simulink model "oversample2x_2samples_per_clock"  (R2016b)
settings: Solver=VariableStepAuto  StartTime=0.0  StopTime=samples_per_channel*number_channels  RelTol=1e-3
PreLoadFcn:
  | setup
values from neighbouring files (symbols this model uses):
  filts = reshape(filt,number_subband,taps_per_chan)    [setup.m]
undefined symbols (not defined in the file or in its folder): j
libraries: dspxfrm3 x8, dspsigops x2
settings Model: Creator=mdewart  LastModifiedBy=mdewart

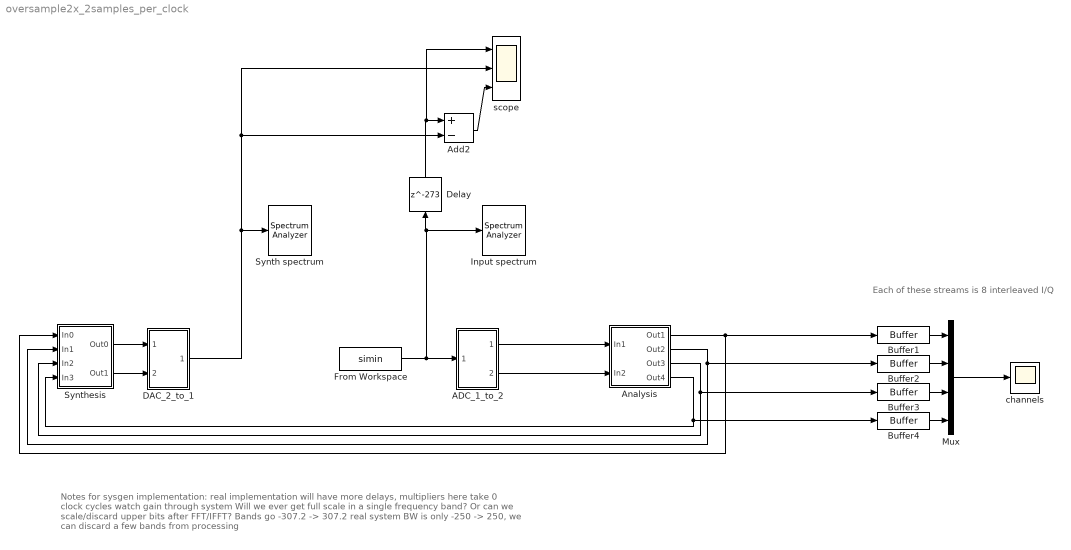
== system oversample2x_2samples_per_clock ==
  note: Notes for sysgen implementation:
      |
      | real implementation will have more delays, multipliers here take 0 clock cycles
      |
      | watch gain through system
      |      Will we ever get full scale in a single frequency band?  Or can we scale/discard upper bits after FFT/IFFT?
      |
      | Bands go -307.2 -> 307.2  real system BW is only -250 -> 250, we can discard a few bands from processing
  note: Each of these streams is 8 interleaved I/Q
  ADC_1_to_2 : Subsystem
  Add2 : Sum  Inputs=+-
  Analysis : Subsystem
  Buffer{1..4} (4 alike) : Buffer  N=8  TreatMby1Signals=One channel  OutputFrames=off
  DAC_2_to_1 : Subsystem
  Delay : Delay  DelayLength=273  InitialCondition=0
  From Workspace : FromWorkspace  VariableName=simin  SampleTime=1  Interpolate=off  OutputAfterFinalValue=Cyclic repetition
  Input spectrum : SpectrumAnalyzer
  Mux : Mux
  Synth spectrum : SpectrumAnalyzer
  Synthesis : Subsystem
  channels : Scope
  scope : Scope  NumInputPorts=3
  wires:
  Synthesis/1(Out0) -> DAC_2_to_1/1(In1)
  Synthesis/2(Out1) -> DAC_2_to_1/2(In2)
  ADC_1_to_2/1(Out1) -> Analysis/1(In1)
  ADC_1_to_2/2(Out2) -> Analysis/2(In2)
  Analysis/4(Out4) -> Buffer4/1, Synthesis/4(In3)
  Analysis/3(Out3) -> Buffer3/1, Synthesis/3(In2)
  Analysis/2(Out2) -> Buffer2/1, Synthesis/2(In1)
  Analysis/1(Out1) -> Buffer1/1, Synthesis/1(In0)
  From Workspace/1 -> Delay/1, Input spectrum/1, ADC_1_to_2/1(In1)
  Mux/1 -> channels/1
  Buffer1/1 -> Mux/1
  Buffer2/1 -> Mux/2
  Buffer3/1 -> Mux/3
  Buffer4/1 -> Mux/4
  Add2/1 -> scope/3
  DAC_2_to_1/1(Out1) -> Add2/2, scope/2, Synth spectrum/1
  Delay/1 -> Add2/1, scope/1

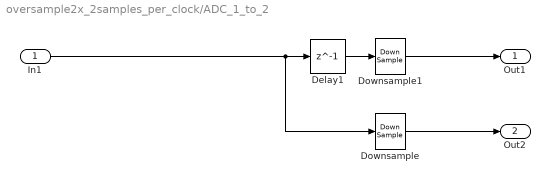
== system oversample2x_2samples_per_clock/ADC_1_to_2 ==
  In1 : Inport
  Delay1 : Delay  DelayLength=1  InitialCondition=0
  Downsample : DownSample  RateOptions=Allow multirate processing
  Downsample1 : DownSample  RateOptions=Allow multirate processing
  Out1 : Outport
  Out2 : Outport  Port=2
  wires:
  Downsample/1 -> Out2/1
  In1/1 -> Downsample/1, Delay1/1
  Downsample1/1 -> Out1/1
  Delay1/1 -> Downsample1/1

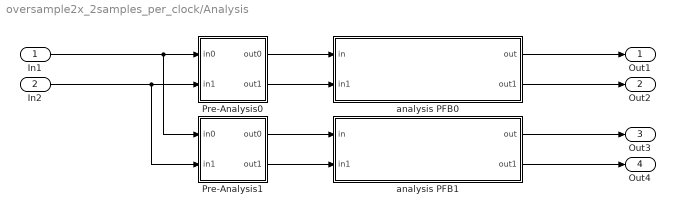
== system oversample2x_2samples_per_clock/Analysis ==
  In1 : Inport
  In2 : Inport  Port=2
  Pre-Analysis0 : Subsystem
  Pre-Analysis1 : Subsystem
  analysis PFB0 : Subsystem
  analysis PFB1 : Subsystem
  Out1 : Outport
  Out2 : Outport  Port=2
  Out3 : Outport  Port=3
  Out4 : Outport  Port=4
  wires:
  analysis PFB0/1(out) -> Out1/1
  analysis PFB1/1(out) -> Out3/1
  Pre-Analysis1/2(out1) -> analysis PFB1/2(in1)
  Pre-Analysis1/1(out0) -> analysis PFB1/1(in)
  Pre-Analysis0/1(out0) -> analysis PFB0/1(in)
  Pre-Analysis0/2(out1) -> analysis PFB0/2(in1)
  analysis PFB1/2(out1) -> Out4/1
  In1/1 -> Pre-Analysis1/1(in0), Pre-Analysis0/1(in0)
  In2/1 -> Pre-Analysis1/2(in1), Pre-Analysis0/2(in1)
  analysis PFB0/2(out1) -> Out2/1

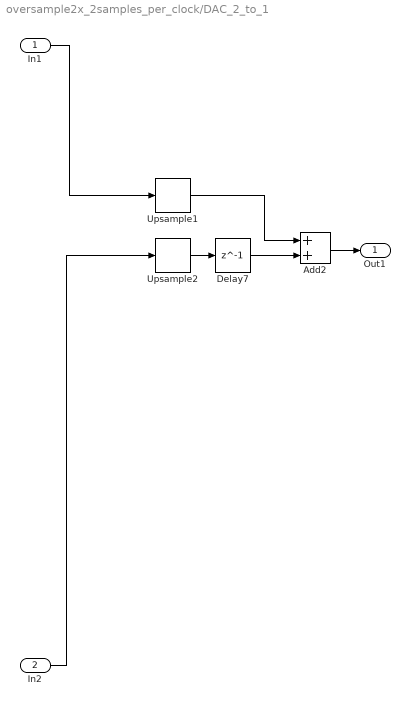
== system oversample2x_2samples_per_clock/DAC_2_to_1 ==
  In1 : Inport
  In2 : Inport  Port=2
  Add2 : Sum
  Delay7 : Delay  DelayLength=1  InitialCondition=0
  Upsample1 : dspsigops/Upsample  N=2  phase=0  RateOptions=Allow multirate processing  ic=0  mode=Unused parameter value
  Upsample2 : dspsigops/Upsample  N=2  phase=0  RateOptions=Allow multirate processing  ic=0  mode=Unused parameter value
  Out1 : Outport
  wires:
  In2/1 -> Upsample2/1
  Delay7/1 -> Add2/2
  In1/1 -> Upsample1/1
  Upsample1/1 -> Add2/1
  Add2/1 -> Out1/1
  Upsample2/1 -> Delay7/1

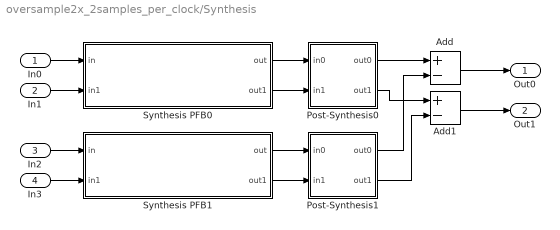
== system oversample2x_2samples_per_clock/Synthesis ==
  In0 : Inport
  In1 : Inport  Port=2
  In2 : Inport  Port=3
  In3 : Inport  Port=4
  Add : Sum  Inputs=+-
  Add1 : Sum  Inputs=+-
  Post-Synthesis0 : Subsystem
  Post-Synthesis1 : Subsystem
  Synthesis PFB0 : Subsystem
  Synthesis PFB1 : Subsystem
  Out0 : Outport
  Out1 : Outport  Port=2
  wires:
  In2/1 -> Synthesis PFB1/1(in)
  In1/1 -> Synthesis PFB0/2(in1)
  In0/1 -> Synthesis PFB0/1(in)
  In3/1 -> Synthesis PFB1/2(in1)
  Synthesis PFB0/2(out1) -> Post-Synthesis0/2(in1)
  Synthesis PFB0/1(out) -> Post-Synthesis0/1(in0)
  Post-Synthesis0/1(out0) -> Add/1
  Post-Synthesis1/1(out0) -> Add/2
  Add/1 -> Out0/1
  Post-Synthesis0/2(out1) -> Add1/1
  Add1/1 -> Out1/1
  Synthesis PFB1/2(out1) -> Post-Synthesis1/2(in1)
  Post-Synthesis1/2(out1) -> Add1/2
  Synthesis PFB1/1(out) -> Post-Synthesis1/1(in0)

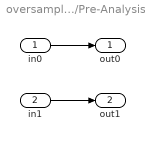
== system oversample2x_2samples_per_clock/Analysis/Pre-Analysis0 ==
  in0 : Inport
  in1 : Inport  Port=2
  out0 : Outport
  out1 : Outport  Port=2
  wires:
  in1/1 -> out1/1
  in0/1 -> out0/1

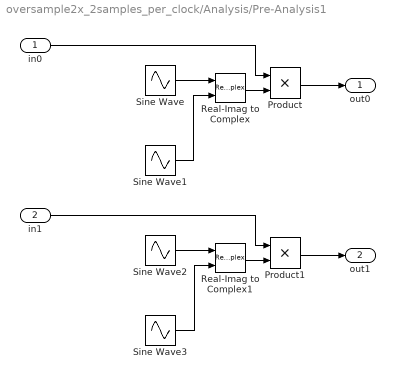
== system oversample2x_2samples_per_clock/Analysis/Pre-Analysis1 ==
  in0 : Inport
  in1 : Inport  Port=2
  Product : Product
  Product1 : Product
  Real-Imag to Complex : RealImagToComplex
  Real-Imag to Complex1 : RealImagToComplex
  Sine Wave : Sin  Frequency=2*pi/32  Phase=-pi/2  SampleTime=2
  Sine Wave1 : Sin  Frequency=2*pi/32  SampleTime=2
  Sine Wave2 : Sin  Frequency=2*pi/32  Phase=-pi/2+pi/16  SampleTime=2
  Sine Wave3 : Sin  Frequency=2*pi/32  Phase=0+pi/16  SampleTime=2
  out0 : Outport
  out1 : Outport  Port=2
  wires:
  in0/1 -> Product/1
  Product/1 -> out0/1
  Product1/1 -> out1/1
  Sine Wave/1 -> Real-Imag to Complex/1
  Sine Wave1/1 -> Real-Imag to Complex/2
  in1/1 -> Product1/1
  Sine Wave2/1 -> Real-Imag to Complex1/1
  Sine Wave3/1 -> Real-Imag to Complex1/2
  Real-Imag to Complex1/1 -> Product1/2
  Real-Imag to Complex/1 -> Product/2

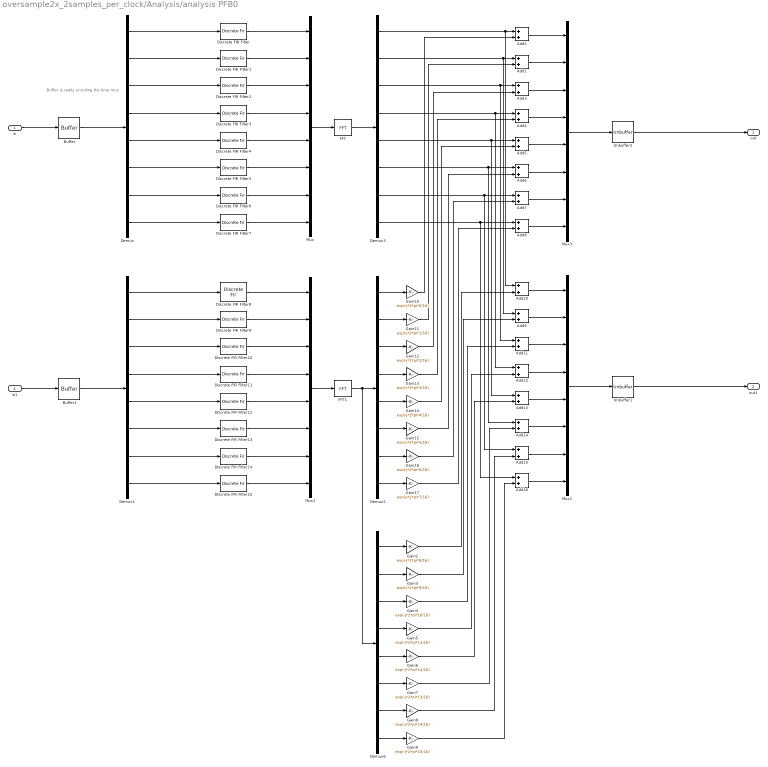
== system oversample2x_2samples_per_clock/Analysis/analysis PFB0 ==
  note: Buffer is really unrolling the time mux
  in : Inport
  in1 : Inport  Port=2
  Add{1..16} (16 alike) : Sum
  Buffer : Buffer  N=8  TreatMby1Signals=One channel  OutputFrames=off
  Buffer1 : Buffer  N=8  TreatMby1Signals=One channel  OutputFrames=off
  Demux{,1..3,6} (5 alike) : Demux  Outputs=8
  Discrete FIR Filter : DiscreteFir  Coefficients=fliplr(filts(1,:))
  Discrete FIR Filter1 : DiscreteFir  Coefficients=fliplr(filts(3,:))
  Discrete FIR Filter10 : DiscreteFir  Coefficients=fliplr(filts(6,:))
  Discrete FIR Filter11 : DiscreteFir  Coefficients=fliplr(filts(8,:))
  Discrete FIR Filter12 : DiscreteFir  Coefficients=fliplr(filts(10,:))
  Discrete FIR Filter13 : DiscreteFir  Coefficients=fliplr(filts(12,:))
  Discrete FIR Filter14 : DiscreteFir  Coefficients=fliplr(filts(14,:))
  Discrete FIR Filter15 : DiscreteFir  Coefficients=fliplr(filts(16,:))
  Discrete FIR Filter2 : DiscreteFir  Coefficients=fliplr(filts(5,:))
  Discrete FIR Filter3 : DiscreteFir  Coefficients=fliplr(filts(7,:))
  Discrete FIR Filter4 : DiscreteFir  Coefficients=fliplr(filts(9,:))
  Discrete FIR Filter5 : DiscreteFir  Coefficients=fliplr(filts(11,:))
  Discrete FIR Filter6 : DiscreteFir  Coefficients=fliplr(filts(13,:))
  Discrete FIR Filter7 : DiscreteFir  Coefficients=fliplr(filts(15,:))
  Discrete FIR Filter8 : DiscreteFir  Coefficients=fliplr(filts(2,:))
  Discrete FIR Filter9 : DiscreteFir  Coefficients=fliplr(filts(4,:))
  FFT : dspxfrm3/FFT  FFTImplementation=Auto  CompMethod=Table lookup  TableOpt=NEW  TableOptActive=Speed  BitRevOrder=off  Normalize=off  InheritFFTLength=on  FFTLength=64  WrapInput=on  roundingMode=Floor  overflowMode=off  firstCoeffDataTypeStr=Inherit: Same word length as input  firstCoeffLastDataTypeStr=Inherit: Same word length as input  outputMin=[]  outputMax=[]
  FFT1 : dspxfrm3/FFT  FFTImplementation=Auto  CompMethod=Table lookup  TableOpt=NEW  TableOptActive=Speed  BitRevOrder=off  Normalize=off  InheritFFTLength=on  FFTLength=64  WrapInput=on  roundingMode=Floor  overflowMode=off  firstCoeffDataTypeStr=Inherit: Same word length as input  firstCoeffLastDataTypeStr=Inherit: Same word length as input  outputMin=[]  outputMax=[]
  Gain10 : Gain  Gain=exp(-j*2*pi*0/16)
  Gain11 : Gain  Gain=exp(-j*2*pi*1/16)
  Gain12 : Gain  Gain=exp(-j*2*pi*2/16)
  Gain13 : Gain  Gain=exp(-j*2*pi*3/16)
  Gain14 : Gain  Gain=exp(-j*2*pi*4/16)
  Gain15 : Gain  Gain=exp(-j*2*pi*5/16)
  Gain16 : Gain  Gain=exp(-j*2*pi*6/16)
  Gain17 : Gain  Gain=exp(-j*2*pi*7/16)
  Gain2 : Gain  Gain=exp(-j*2*pi*8/16)
  Gain3 : Gain  Gain=exp(-j*2*pi*9/16)
  Gain4 : Gain  Gain=exp(-j*2*pi*10/16)
  Gain5 : Gain  Gain=exp(-j*2*pi*11/16)
  Gain6 : Gain  Gain=exp(-j*2*pi*12/16)
  Gain7 : Gain  Gain=exp(-j*2*pi*13/16)
  Gain8 : Gain  Gain=exp(-j*2*pi*14/16)
  Gain9 : Gain  Gain=exp(-j*2*pi*15/16)
  Mux{,1..3} (4 alike) : Mux  Inputs=8
  Unbuffer1 : Unbuffer  SampleBasedProcessing=Same as frame based
  Unbuffer2 : Unbuffer  SampleBasedProcessing=Same as frame based
  out : Outport
  out1 : Outport  Port=2
  wires:
  Add16/1 -> Mux2/8
  Add15/1 -> Mux2/7
  Demux2/2 -> Gain11/1
  Demux2/6 -> Gain15/1
  Demux2/3 -> Gain12/1
  Demux2/5 -> Gain14/1
  Demux2/1 -> Gain10/1
  Demux2/8 -> Gain17/1
  Demux2/7 -> Gain16/1
  Demux2/4 -> Gain13/1
  Mux1/1 -> FFT1/1
  Demux1/4 -> Discrete FIR Filter11/1
  Discrete FIR Filter14/1 -> Mux1/7
  Discrete FIR Filter11/1 -> Mux1/4
  Discrete FIR Filter9/1 -> Mux1/2
  Discrete FIR Filter10/1 -> Mux1/3
  Discrete FIR Filter12/1 -> Mux1/5
  Discrete FIR Filter8/1 -> Mux1/1
  Discrete FIR Filter13/1 -> Mux1/6
  Demux1/6 -> Discrete FIR Filter13/1
  Demux1/1 -> Discrete FIR Filter8/1
  Demux1/3 -> Discrete FIR Filter10/1
  Demux1/8 -> Discrete FIR Filter15/1
  Demux1/5 -> Discrete FIR Filter12/1
  Demux1/7 -> Discrete FIR Filter14/1
  Demux1/2 -> Discrete FIR Filter9/1
  Discrete FIR Filter15/1 -> Mux1/8
  Mux/1 -> FFT/1
  Demux/4 -> Discrete FIR Filter3/1
  Discrete FIR Filter6/1 -> Mux/7
  Discrete FIR Filter3/1 -> Mux/4
  Discrete FIR Filter1/1 -> Mux/2
  Discrete FIR Filter2/1 -> Mux/3
  Discrete FIR Filter4/1 -> Mux/5
  Discrete FIR Filter/1 -> Mux/1
  Discrete FIR Filter5/1 -> Mux/6
  Demux/6 -> Discrete FIR Filter5/1
  Demux/1 -> Discrete FIR Filter/1
  Demux/3 -> Discrete FIR Filter2/1
  Demux/8 -> Discrete FIR Filter7/1
  Demux/5 -> Discrete FIR Filter4/1
  Demux/7 -> Discrete FIR Filter6/1
  Demux/2 -> Discrete FIR Filter1/1
  Buffer/1 -> Demux/1
  Discrete FIR Filter7/1 -> Mux/8
  Buffer1/1 -> Demux1/1
  Mux2/1 -> Unbuffer1/1
  Unbuffer2/1 -> out/1
  FFT/1 -> Demux3/1
  Demux3/8 -> Add16/1, Add8/1
  Demux3/7 -> Add15/1, Add7/1
  Demux3/6 -> Add14/1, Add6/1
  Demux3/5 -> Add13/1, Add5/1
  Demux3/4 -> Add12/1, Add4/1
  Demux3/3 -> Add11/1, Add3/1
  Demux3/2 -> Add9/1, Add1/1
  Demux3/1 -> Add10/1, Add2/1
  Add2/1 -> Mux3/1
  Add1/1 -> Mux3/2
  Add5/1 -> Mux3/5
  Add6/1 -> Mux3/6
  Add3/1 -> Mux3/3
  Add7/1 -> Mux3/7
  Add4/1 -> Mux3/4
  Add8/1 -> Mux3/8
  Mux3/1 -> Unbuffer2/1
  in/1 -> Buffer/1
  Add10/1 -> Mux2/1
  Add11/1 -> Mux2/3
  Add12/1 -> Mux2/4
  Add13/1 -> Mux2/5
  Add14/1 -> Mux2/6
  Add9/1 -> Mux2/2
  Unbuffer1/1 -> out1/1
  Gain10/1 -> Add2/2
  Gain11/1 -> Add1/2
  Gain12/1 -> Add3/2
  Gain13/1 -> Add4/2
  Gain14/1 -> Add5/2
  Gain15/1 -> Add6/2
  Gain16/1 -> Add7/2
  Gain17/1 -> Add8/2
  Demux6/2 -> Gain3/1
  Demux6/6 -> Gain7/1
  Demux6/3 -> Gain4/1
  Demux6/5 -> Gain6/1
  Demux6/1 -> Gain2/1
  Demux6/8 -> Gain9/1
  Demux6/7 -> Gain8/1
  Demux6/4 -> Gain5/1
  FFT1/1 -> Demux6/1, Demux2/1
  Gain2/1 -> Add10/2
  Gain3/1 -> Add9/2
  Gain4/1 -> Add11/2
  Gain5/1 -> Add12/2
  Gain6/1 -> Add13/2
  Gain7/1 -> Add14/2
  Gain8/1 -> Add15/2
  Gain9/1 -> Add16/2
  in1/1 -> Buffer1/1

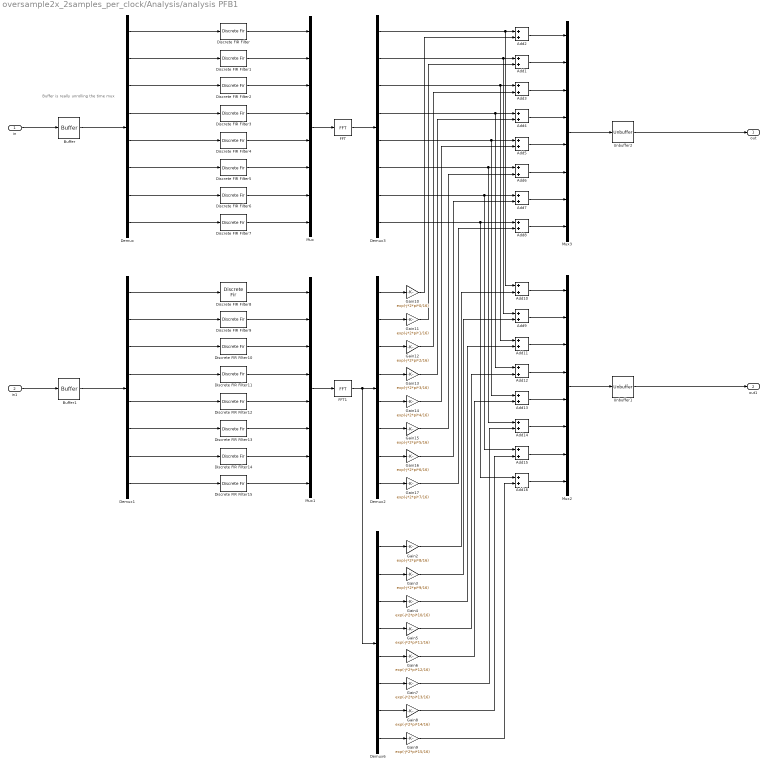
== system oversample2x_2samples_per_clock/Analysis/analysis PFB1 ==
  note: Buffer is really unrolling the time mux
  in : Inport
  in1 : Inport  Port=2
  Add{1..16} (16 alike) : Sum
  Buffer : Buffer  N=8  TreatMby1Signals=One channel  OutputFrames=off
  Buffer1 : Buffer  N=8  TreatMby1Signals=One channel  OutputFrames=off
  Demux{,1..3,6} (5 alike) : Demux  Outputs=8
  Discrete FIR Filter : DiscreteFir  Coefficients=fliplr(filts(1,:))
  Discrete FIR Filter1 : DiscreteFir  Coefficients=fliplr(filts(3,:))
  Discrete FIR Filter10 : DiscreteFir  Coefficients=fliplr(filts(6,:))
  Discrete FIR Filter11 : DiscreteFir  Coefficients=fliplr(filts(8,:))
  Discrete FIR Filter12 : DiscreteFir  Coefficients=fliplr(filts(10,:))
  Discrete FIR Filter13 : DiscreteFir  Coefficients=fliplr(filts(12,:))
  Discrete FIR Filter14 : DiscreteFir  Coefficients=fliplr(filts(14,:))
  Discrete FIR Filter15 : DiscreteFir  Coefficients=fliplr(filts(16,:))
  Discrete FIR Filter2 : DiscreteFir  Coefficients=fliplr(filts(5,:))
  Discrete FIR Filter3 : DiscreteFir  Coefficients=fliplr(filts(7,:))
  Discrete FIR Filter4 : DiscreteFir  Coefficients=fliplr(filts(9,:))
  Discrete FIR Filter5 : DiscreteFir  Coefficients=fliplr(filts(11,:))
  Discrete FIR Filter6 : DiscreteFir  Coefficients=fliplr(filts(13,:))
  Discrete FIR Filter7 : DiscreteFir  Coefficients=fliplr(filts(15,:))
  Discrete FIR Filter8 : DiscreteFir  Coefficients=fliplr(filts(2,:))
  Discrete FIR Filter9 : DiscreteFir  Coefficients=fliplr(filts(4,:))
  FFT : dspxfrm3/FFT  FFTImplementation=Auto  CompMethod=Table lookup  TableOpt=NEW  TableOptActive=Speed  BitRevOrder=off  Normalize=off  InheritFFTLength=on  FFTLength=64  WrapInput=on  roundingMode=Floor  overflowMode=off  firstCoeffDataTypeStr=Inherit: Same word length as input  firstCoeffLastDataTypeStr=Inherit: Same word length as input  outputMin=[]  outputMax=[]
  FFT1 : dspxfrm3/FFT  FFTImplementation=Auto  CompMethod=Table lookup  TableOpt=NEW  TableOptActive=Speed  BitRevOrder=off  Normalize=off  InheritFFTLength=on  FFTLength=64  WrapInput=on  roundingMode=Floor  overflowMode=off  firstCoeffDataTypeStr=Inherit: Same word length as input  firstCoeffLastDataTypeStr=Inherit: Same word length as input  outputMin=[]  outputMax=[]
  Gain10 : Gain  Gain=exp(-j*2*pi*0/16)
  Gain11 : Gain  Gain=exp(-j*2*pi*1/16)
  Gain12 : Gain  Gain=exp(-j*2*pi*2/16)
  Gain13 : Gain  Gain=exp(-j*2*pi*3/16)
  Gain14 : Gain  Gain=exp(-j*2*pi*4/16)
  Gain15 : Gain  Gain=exp(-j*2*pi*5/16)
  Gain16 : Gain  Gain=exp(-j*2*pi*6/16)
  Gain17 : Gain  Gain=exp(-j*2*pi*7/16)
  Gain2 : Gain  Gain=exp(-j*2*pi*8/16)
  Gain3 : Gain  Gain=exp(-j*2*pi*9/16)
  Gain4 : Gain  Gain=exp(-j*2*pi*10/16)
  Gain5 : Gain  Gain=exp(-j*2*pi*11/16)
  Gain6 : Gain  Gain=exp(-j*2*pi*12/16)
  Gain7 : Gain  Gain=exp(-j*2*pi*13/16)
  Gain8 : Gain  Gain=exp(-j*2*pi*14/16)
  Gain9 : Gain  Gain=exp(-j*2*pi*15/16)
  Mux{,1..3} (4 alike) : Mux  Inputs=8
  Unbuffer1 : Unbuffer  SampleBasedProcessing=Same as frame based
  Unbuffer2 : Unbuffer  SampleBasedProcessing=Same as frame based
  out : Outport
  out1 : Outport  Port=2
  wires:
  in1/1 -> Buffer1/1
  Gain9/1 -> Add16/2
  Gain8/1 -> Add15/2
  Gain7/1 -> Add14/2
  Gain6/1 -> Add13/2
  Gain5/1 -> Add12/2
  Gain4/1 -> Add11/2
  Gain3/1 -> Add9/2
  Gain2/1 -> Add10/2
  FFT1/1 -> Demux2/1, Demux6/1
  Demux6/4 -> Gain5/1
  Demux6/7 -> Gain8/1
  Demux6/8 -> Gain9/1
  Demux6/1 -> Gain2/1
  Demux6/5 -> Gain6/1
  Demux6/3 -> Gain4/1
  Demux6/6 -> Gain7/1
  Demux6/2 -> Gain3/1
  Gain17/1 -> Add8/2
  Gain16/1 -> Add7/2
  Gain15/1 -> Add6/2
  Gain14/1 -> Add5/2
  Gain13/1 -> Add4/2
  Gain12/1 -> Add3/2
  Gain11/1 -> Add1/2
  Gain10/1 -> Add2/2
  Unbuffer1/1 -> out1/1
  Add9/1 -> Mux2/2
  Add14/1 -> Mux2/6
  Add13/1 -> Mux2/5
  Add12/1 -> Mux2/4
  Add11/1 -> Mux2/3
  Add10/1 -> Mux2/1
  in/1 -> Buffer/1
  Mux3/1 -> Unbuffer2/1
  Add8/1 -> Mux3/8
  Add4/1 -> Mux3/4
  Add7/1 -> Mux3/7
  Add3/1 -> Mux3/3
  Add6/1 -> Mux3/6
  Add5/1 -> Mux3/5
  Add1/1 -> Mux3/2
  Add2/1 -> Mux3/1
  Demux3/1 -> Add2/1, Add10/1
  Demux3/2 -> Add1/1, Add9/1
  Demux3/3 -> Add3/1, Add11/1
  Demux3/4 -> Add4/1, Add12/1
  Demux3/5 -> Add5/1, Add13/1
  Demux3/6 -> Add6/1, Add14/1
  Demux3/7 -> Add7/1, Add15/1
  Demux3/8 -> Add8/1, Add16/1
  FFT/1 -> Demux3/1
  Unbuffer2/1 -> out/1
  Mux2/1 -> Unbuffer1/1
  Buffer1/1 -> Demux1/1
  Discrete FIR Filter7/1 -> Mux/8
  Buffer/1 -> Demux/1
  Demux/2 -> Discrete FIR Filter1/1
  Demux/7 -> Discrete FIR Filter6/1
  Demux/5 -> Discrete FIR Filter4/1
  Demux/8 -> Discrete FIR Filter7/1
  Demux/3 -> Discrete FIR Filter2/1
  Demux/1 -> Discrete FIR Filter/1
  Demux/6 -> Discrete FIR Filter5/1
  Discrete FIR Filter5/1 -> Mux/6
  Discrete FIR Filter/1 -> Mux/1
  Discrete FIR Filter4/1 -> Mux/5
  Discrete FIR Filter2/1 -> Mux/3
  Discrete FIR Filter1/1 -> Mux/2
  Discrete FIR Filter3/1 -> Mux/4
  Discrete FIR Filter6/1 -> Mux/7
  Demux/4 -> Discrete FIR Filter3/1
  Mux/1 -> FFT/1
  Discrete FIR Filter15/1 -> Mux1/8
  Demux1/2 -> Discrete FIR Filter9/1
  Demux1/7 -> Discrete FIR Filter14/1
  Demux1/5 -> Discrete FIR Filter12/1
  Demux1/8 -> Discrete FIR Filter15/1
  Demux1/3 -> Discrete FIR Filter10/1
  Demux1/1 -> Discrete FIR Filter8/1
  Demux1/6 -> Discrete FIR Filter13/1
  Discrete FIR Filter13/1 -> Mux1/6
  Discrete FIR Filter8/1 -> Mux1/1
  Discrete FIR Filter12/1 -> Mux1/5
  Discrete FIR Filter10/1 -> Mux1/3
  Discrete FIR Filter9/1 -> Mux1/2
  Discrete FIR Filter11/1 -> Mux1/4
  Discrete FIR Filter14/1 -> Mux1/7
  Demux1/4 -> Discrete FIR Filter11/1
  Mux1/1 -> FFT1/1
  Demux2/4 -> Gain13/1
  Demux2/7 -> Gain16/1
  Demux2/8 -> Gain17/1
  Demux2/1 -> Gain10/1
  Demux2/5 -> Gain14/1
  Demux2/3 -> Gain12/1
  Demux2/6 -> Gain15/1
  Demux2/2 -> Gain11/1
  Add15/1 -> Mux2/7
  Add16/1 -> Mux2/8

== system oversample2x_2samples_per_clock/Synthesis/Post-Synthesis0 ==
  note: Post-synthesis0 match timing to post-synthesis
  in0 : Inport
  in1 : Inport  Port=2
  out0 : Outport
  out1 : Outport  Port=2
  wires:
  in1/1 -> out1/1
  in0/1 -> out0/1

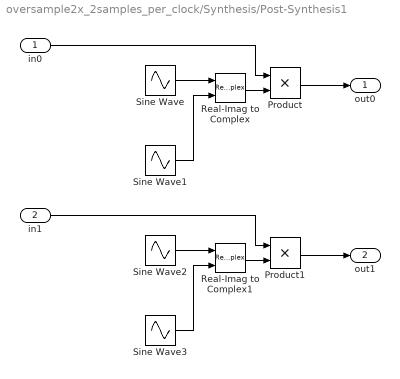
== system oversample2x_2samples_per_clock/Synthesis/Post-Synthesis1 ==
  in0 : Inport
  in1 : Inport  Port=2
  Product : Product
  Product1 : Product
  Real-Imag to Complex : RealImagToComplex
  Real-Imag to Complex1 : RealImagToComplex
  Sine Wave : Sin  Frequency=2*pi/32  Phase=-pi/2  SampleTime=2
  Sine Wave1 : Sin  Amplitude=-1  Frequency=2*pi/32  SampleTime=2
  Sine Wave2 : Sin  Frequency=2*pi/32  Phase=-pi/2+pi/16  SampleTime=2
  Sine Wave3 : Sin  Amplitude=-1  Frequency=2*pi/32  Phase=0+pi/16  SampleTime=2
  out0 : Outport
  out1 : Outport  Port=2
  wires:
  in0/1 -> Product/1
  ? -> ?
  ? -> ?
  Product/1 -> out0/1
  Product1/1 -> out1/1
  Sine Wave/1 -> Real-Imag to Complex/1
  Sine Wave1/1 -> Real-Imag to Complex/2
  in1/1 -> Product1/1
  Sine Wave2/1 -> Real-Imag to Complex1/1
  Sine Wave3/1 -> Real-Imag to Complex1/2
  Real-Imag to Complex1/1 -> Product1/2
  Real-Imag to Complex/1 -> Product/2

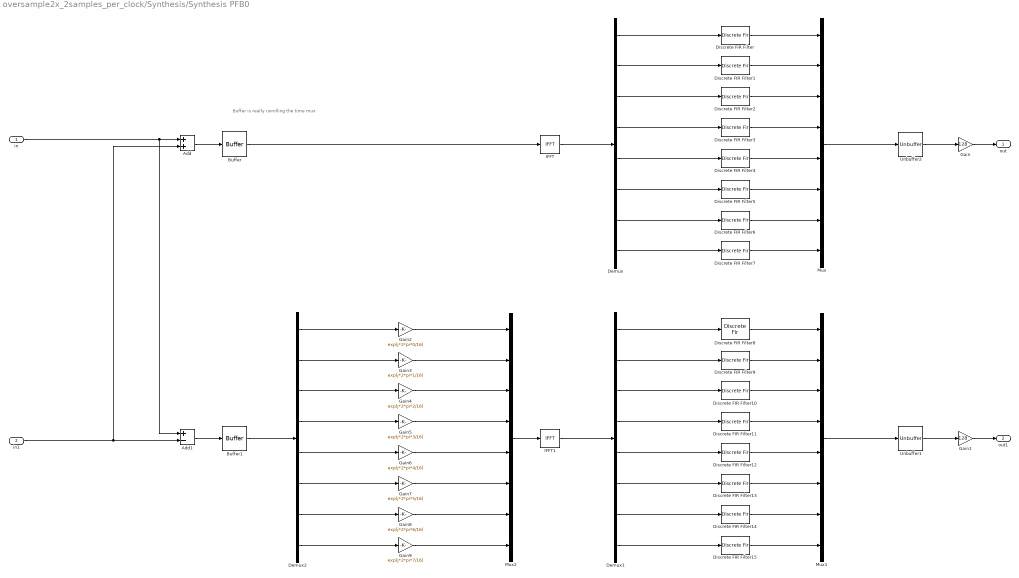
== system oversample2x_2samples_per_clock/Synthesis/Synthesis PFB0 ==
  note: Buffer is really unrolling the time mux
  in : Inport
  in1 : Inport  Port=2
  Add : Sum
  Add1 : Sum  Inputs=+-
  Buffer : Buffer  N=8  TreatMby1Signals=One channel  OutputFrames=off
  Buffer1 : Buffer  N=8  TreatMby1Signals=One channel  OutputFrames=off
  Demux : Demux  Outputs=8
  Demux1 : Demux  Outputs=8
  Demux2 : Demux  Outputs=8
  Discrete FIR Filter : DiscreteFir  Coefficients=filts(1,:)
  Discrete FIR Filter1 : DiscreteFir  Coefficients=filts(3,:)
  Discrete FIR Filter10 : DiscreteFir  Coefficients=filts(6,:)
  Discrete FIR Filter11 : DiscreteFir  Coefficients=filts(8,:)
  Discrete FIR Filter12 : DiscreteFir  Coefficients=filts(10,:)
  Discrete FIR Filter13 : DiscreteFir  Coefficients=filts(12,:)
  Discrete FIR Filter14 : DiscreteFir  Coefficients=filts(14,:)
  Discrete FIR Filter15 : DiscreteFir  Coefficients=filts(16,:)
  Discrete FIR Filter2 : DiscreteFir  Coefficients=filts(5,:)
  Discrete FIR Filter3 : DiscreteFir  Coefficients=filts(7,:)
  Discrete FIR Filter4 : DiscreteFir  Coefficients=filts(9,:)
  Discrete FIR Filter5 : DiscreteFir  Coefficients=filts(11,:)
  Discrete FIR Filter6 : DiscreteFir  Coefficients=filts(13,:)
  Discrete FIR Filter7 : DiscreteFir  Coefficients=filts(15,:)
  Discrete FIR Filter8 : DiscreteFir  Coefficients=filts(2,:)
  Discrete FIR Filter9 : DiscreteFir  Coefficients=filts(4,:)
  Gain : Gain  Gain=128
  Gain1 : Gain  Gain=128
  Gain2 : Gain  Gain=exp(j*2*pi*0/16)
  Gain3 : Gain  Gain=exp(j*2*pi*1/16)
  Gain4 : Gain  Gain=exp(j*2*pi*2/16)
  Gain5 : Gain  Gain=exp(j*2*pi*3/16)
  Gain6 : Gain  Gain=exp(j*2*pi*4/16)
  Gain7 : Gain  Gain=exp(j*2*pi*5/16)
  Gain8 : Gain  Gain=exp(j*2*pi*6/16)
  Gain9 : Gain  Gain=exp(j*2*pi*7/16)
  IFFT : dspxfrm3/IFFT  FFTImplementation=Auto  CompMethod=Table lookup  TableOpt=NEW  TableOptActive=Speed  BitRevOrder=off  cs_in=off  Normalize=on  InheritFFTLength=on  FFTLength=64  WrapInput=on  mode=Complex  outSamplingMode=Sample based  roundingMode=Floor  overflowMode=off  firstCoeffDataTypeStr=Inherit: Same word length as input  firstCoeffLastDataTypeStr=Inherit: Same word length as input  outputMin=[]  outputMax=[]
  IFFT1 : dspxfrm3/IFFT  FFTImplementation=Auto  CompMethod=Table lookup  TableOpt=NEW  TableOptActive=Speed  BitRevOrder=off  cs_in=off  Normalize=on  InheritFFTLength=on  FFTLength=64  WrapInput=on  mode=Complex  outSamplingMode=Sample based  roundingMode=Floor  overflowMode=off  firstCoeffDataTypeStr=Inherit: Same word length as input  firstCoeffLastDataTypeStr=Inherit: Same word length as input  outputMin=[]  outputMax=[]
  Mux : Mux  Inputs=8
  Mux1 : Mux  Inputs=8
  Mux2 : Mux  Inputs=8
  Unbuffer1 : Unbuffer  SampleBasedProcessing=Same as frame based
  Unbuffer2 : Unbuffer  SampleBasedProcessing=Same as frame based
  out : Outport
  out1 : Outport  Port=2
  wires:
  Discrete FIR Filter7/1 -> Mux/8
  IFFT/1 -> Demux/1
  Demux/2 -> Discrete FIR Filter1/1
  Demux/7 -> Discrete FIR Filter6/1
  Demux/5 -> Discrete FIR Filter4/1
  Demux/8 -> Discrete FIR Filter7/1
  Demux/3 -> Discrete FIR Filter2/1
  Demux/1 -> Discrete FIR Filter/1
  Demux/6 -> Discrete FIR Filter5/1
  Discrete FIR Filter5/1 -> Mux/6
  Discrete FIR Filter/1 -> Mux/1
  Discrete FIR Filter4/1 -> Mux/5
  Discrete FIR Filter2/1 -> Mux/3
  Discrete FIR Filter1/1 -> Mux/2
  Discrete FIR Filter3/1 -> Mux/4
  Discrete FIR Filter6/1 -> Mux/7
  Demux/4 -> Discrete FIR Filter3/1
  Mux/1 -> Unbuffer2/1
  Unbuffer2/1 -> Gain/1
  Add/1 -> Buffer/1
  in/1 -> Add1/1, Add/1
  Discrete FIR Filter15/1 -> Mux1/8
  IFFT1/1 -> Demux1/1
  Demux1/2 -> Discrete FIR Filter9/1
  Demux1/7 -> Discrete FIR Filter14/1
  Demux1/5 -> Discrete FIR Filter12/1
  Demux1/8 -> Discrete FIR Filter15/1
  Demux1/3 -> Discrete FIR Filter10/1
  Demux1/1 -> Discrete FIR Filter8/1
  Demux1/6 -> Discrete FIR Filter13/1
  Discrete FIR Filter13/1 -> Mux1/6
  Discrete FIR Filter8/1 -> Mux1/1
  Discrete FIR Filter12/1 -> Mux1/5
  Discrete FIR Filter10/1 -> Mux1/3
  Discrete FIR Filter9/1 -> Mux1/2
  Discrete FIR Filter11/1 -> Mux1/4
  Discrete FIR Filter14/1 -> Mux1/7
  Demux1/4 -> Discrete FIR Filter11/1
  Mux1/1 -> Unbuffer1/1
  Unbuffer1/1 -> Gain1/1
  Add1/1 -> Buffer1/1
  in1/1 -> Add/2, Add1/2
  Mux2/1 -> IFFT1/1
  Demux2/4 -> Gain5/1
  Demux2/7 -> Gain8/1
  Demux2/8 -> Gain9/1
  Demux2/1 -> Gain2/1
  Demux2/5 -> Gain6/1
  Demux2/3 -> Gain4/1
  Demux2/6 -> Gain7/1
  Demux2/2 -> Gain3/1
  Gain2/1 -> Mux2/1
  Gain3/1 -> Mux2/2
  Gain4/1 -> Mux2/3
  Gain5/1 -> Mux2/4
  Gain6/1 -> Mux2/5
  Gain7/1 -> Mux2/6
  Gain8/1 -> Mux2/7
  Gain9/1 -> Mux2/8
  Gain/1 -> out/1
  Gain1/1 -> out1/1
  Buffer/1 -> IFFT/1
  Buffer1/1 -> Demux2/1

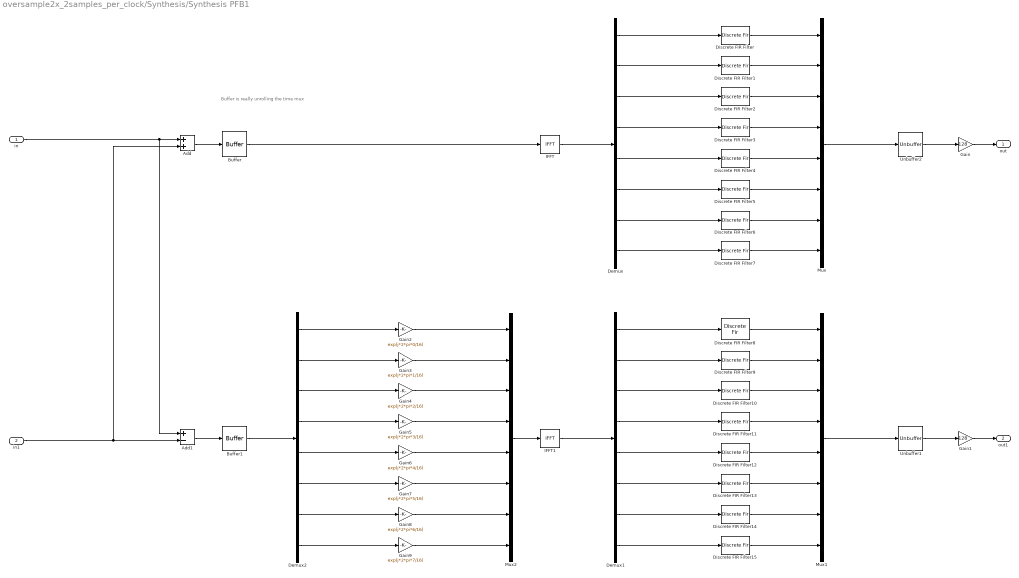
== system oversample2x_2samples_per_clock/Synthesis/Synthesis PFB1 ==
  note: Buffer is really unrolling the time mux
  in : Inport
  in1 : Inport  Port=2
  Add : Sum
  Add1 : Sum  Inputs=+-
  Buffer : Buffer  N=8  TreatMby1Signals=One channel  OutputFrames=off
  Buffer1 : Buffer  N=8  TreatMby1Signals=One channel  OutputFrames=off
  Demux : Demux  Outputs=8
  Demux1 : Demux  Outputs=8
  Demux2 : Demux  Outputs=8
  Discrete FIR Filter : DiscreteFir  Coefficients=filts(1,:)
  Discrete FIR Filter1 : DiscreteFir  Coefficients=filts(3,:)
  Discrete FIR Filter10 : DiscreteFir  Coefficients=filts(6,:)
  Discrete FIR Filter11 : DiscreteFir  Coefficients=filts(8,:)
  Discrete FIR Filter12 : DiscreteFir  Coefficients=filts(10,:)
  Discrete FIR Filter13 : DiscreteFir  Coefficients=filts(12,:)
  Discrete FIR Filter14 : DiscreteFir  Coefficients=filts(14,:)
  Discrete FIR Filter15 : DiscreteFir  Coefficients=filts(16,:)
  Discrete FIR Filter2 : DiscreteFir  Coefficients=filts(5,:)
  Discrete FIR Filter3 : DiscreteFir  Coefficients=filts(7,:)
  Discrete FIR Filter4 : DiscreteFir  Coefficients=filts(9,:)
  Discrete FIR Filter5 : DiscreteFir  Coefficients=filts(11,:)
  Discrete FIR Filter6 : DiscreteFir  Coefficients=filts(13,:)
  Discrete FIR Filter7 : DiscreteFir  Coefficients=filts(15,:)
  Discrete FIR Filter8 : DiscreteFir  Coefficients=filts(2,:)
  Discrete FIR Filter9 : DiscreteFir  Coefficients=filts(4,:)
  Gain : Gain  Gain=128
  Gain1 : Gain  Gain=128
  Gain2 : Gain  Gain=exp(j*2*pi*0/16)
  Gain3 : Gain  Gain=exp(j*2*pi*1/16)
  Gain4 : Gain  Gain=exp(j*2*pi*2/16)
  Gain5 : Gain  Gain=exp(j*2*pi*3/16)
  Gain6 : Gain  Gain=exp(j*2*pi*4/16)
  Gain7 : Gain  Gain=exp(j*2*pi*5/16)
  Gain8 : Gain  Gain=exp(j*2*pi*6/16)
  Gain9 : Gain  Gain=exp(j*2*pi*7/16)
  IFFT : dspxfrm3/IFFT  FFTImplementation=Auto  CompMethod=Table lookup  TableOpt=NEW  TableOptActive=Speed  BitRevOrder=off  cs_in=off  Normalize=on  InheritFFTLength=on  FFTLength=64  WrapInput=on  mode=Complex  outSamplingMode=Sample based  roundingMode=Floor  overflowMode=off  firstCoeffDataTypeStr=Inherit: Same word length as input  firstCoeffLastDataTypeStr=Inherit: Same word length as input  outputMin=[]  outputMax=[]
  IFFT1 : dspxfrm3/IFFT  FFTImplementation=Auto  CompMethod=Table lookup  TableOpt=NEW  TableOptActive=Speed  BitRevOrder=off  cs_in=off  Normalize=on  InheritFFTLength=on  FFTLength=64  WrapInput=on  mode=Complex  outSamplingMode=Sample based  roundingMode=Floor  overflowMode=off  firstCoeffDataTypeStr=Inherit: Same word length as input  firstCoeffLastDataTypeStr=Inherit: Same word length as input  outputMin=[]  outputMax=[]
  Mux : Mux  Inputs=8
  Mux1 : Mux  Inputs=8
  Mux2 : Mux  Inputs=8
  Unbuffer1 : Unbuffer  SampleBasedProcessing=Same as frame based
  Unbuffer2 : Unbuffer  SampleBasedProcessing=Same as frame based
  out : Outport
  out1 : Outport  Port=2
  wires:
  Discrete FIR Filter7/1 -> Mux/8
  IFFT/1 -> Demux/1
  Demux/2 -> Discrete FIR Filter1/1
  Demux/7 -> Discrete FIR Filter6/1
  Demux/5 -> Discrete FIR Filter4/1
  Demux/8 -> Discrete FIR Filter7/1
  Demux/3 -> Discrete FIR Filter2/1
  Demux/1 -> Discrete FIR Filter/1
  Demux/6 -> Discrete FIR Filter5/1
  Discrete FIR Filter5/1 -> Mux/6
  Discrete FIR Filter/1 -> Mux/1
  Discrete FIR Filter4/1 -> Mux/5
  Discrete FIR Filter2/1 -> Mux/3
  Discrete FIR Filter1/1 -> Mux/2
  Discrete FIR Filter3/1 -> Mux/4
  Discrete FIR Filter6/1 -> Mux/7
  Demux/4 -> Discrete FIR Filter3/1
  Mux/1 -> Unbuffer2/1
  Unbuffer2/1 -> Gain/1
  Add/1 -> Buffer/1
  in/1 -> Add1/1, Add/1
  Discrete FIR Filter15/1 -> Mux1/8
  IFFT1/1 -> Demux1/1
  Demux1/2 -> Discrete FIR Filter9/1
  Demux1/7 -> Discrete FIR Filter14/1
  Demux1/5 -> Discrete FIR Filter12/1
  Demux1/8 -> Discrete FIR Filter15/1
  Demux1/3 -> Discrete FIR Filter10/1
  Demux1/1 -> Discrete FIR Filter8/1
  Demux1/6 -> Discrete FIR Filter13/1
  Discrete FIR Filter13/1 -> Mux1/6
  Discrete FIR Filter8/1 -> Mux1/1
  Discrete FIR Filter12/1 -> Mux1/5
  Discrete FIR Filter10/1 -> Mux1/3
  Discrete FIR Filter9/1 -> Mux1/2
  Discrete FIR Filter11/1 -> Mux1/4
  Discrete FIR Filter14/1 -> Mux1/7
  Demux1/4 -> Discrete FIR Filter11/1
  Mux1/1 -> Unbuffer1/1
  Unbuffer1/1 -> Gain1/1
  Add1/1 -> Buffer1/1
  in1/1 -> Add/2, Add1/2
  Mux2/1 -> IFFT1/1
  Demux2/4 -> Gain5/1
  Demux2/7 -> Gain8/1
  Demux2/8 -> Gain9/1
  Demux2/1 -> Gain2/1
  Demux2/5 -> Gain6/1
  Demux2/3 -> Gain4/1
  Demux2/6 -> Gain7/1
  Demux2/2 -> Gain3/1
  Gain2/1 -> Mux2/1
  Gain3/1 -> Mux2/2
  Gain4/1 -> Mux2/3
  Gain5/1 -> Mux2/4
  Gain6/1 -> Mux2/5
  Gain7/1 -> Mux2/6
  Gain8/1 -> Mux2/7
  Gain9/1 -> Mux2/8
  Gain/1 -> out/1
  Gain1/1 -> out1/1
  Buffer/1 -> IFFT/1
  Buffer1/1 -> Demux2/1
